simulink model "BLOC_Auxiliary_network_12V"  (R2016a)
settings: Solver=VariableStepAuto  StartTime=0.0  StopTime=10.0  RelTol=1e-3
undefined symbols (not defined in the file): hev_dt, syse_aux_current, syse_aux_voltage, syse_dcdc_efficency, syse_dcdc_in_power
settings Model: Creator=Florent  LastModifiedBy=Florent
settings OptimizationCC: DefaultParameterBehavior=Inlined  OptimizeModelRefInitCode=on  LifeSpan=1
settings RTWCC: SystemTargetFile=ert.tlc  TemplateMakefile=ert_default_tmf  GenerateReport=on  IncludeHyperlinkInReport=on  LaunchReport=on  TargetLang=C++  GenerateTraceInfo=on  GenerateTraceReport=on  GenerateTraceReportSl=on  GenerateTraceReportSf=on  GenerateTraceReportEml=on
settings CodeAppCC: ForceParamTrailComments=on  OperatorAnnotations=on  SimulinkDataObjDesc=on  SFDataObjDesc=on  MATLABFcnDesc=on  InsertBlockDesc=on  MATLABSourceComments=on
settings ERTTargetCC: GenerateSampleERTMain=on  MultiInstanceERTCode=on  CodeInterfacePackaging=C++ class  InlinedParameterPlacement=NonHierarchical  RootIOFormat=Structure reference  ERTCustomFileTemplate=example_file_process.tlc

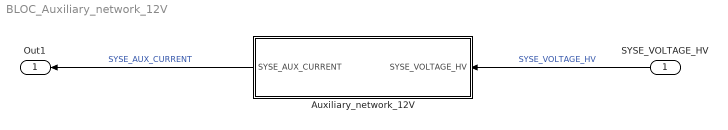
== system BLOC_Auxiliary_network_12V ==
  SYSE_VOLTAGE_HV : Inport
  Auxiliary_network_12V : Subsystem  TreatAsAtomicUnit=on  SystemSampleTime=hev_dt
  Out1 : Outport
  wires:
  Auxiliary_network_12V/1(SYSE_AUX_CURRENT) -> Out1/1  "SYSE_AUX_CURRENT"
  SYSE_VOLTAGE_HV/1 -> Auxiliary_network_12V/1(SYSE_VOLTAGE_HV)  "SYSE_VOLTAGE_HV"

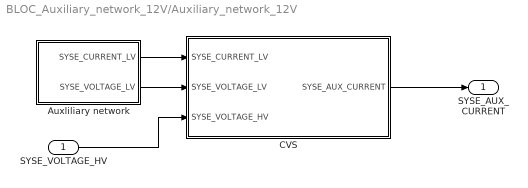
== system BLOC_Auxiliary_network_12V/Auxiliary_network_12V ==
  SYSE_VOLTAGE_HV : Inport
  Auxliliary network : Subsystem
  CVS : Subsystem
  SYSE_AUX_CURRENT : Outport
  wires:
  Auxliliary network/1(SYSE_CURRENT_LV) -> CVS/1(SYSE_CURRENT_LV)
  Auxliliary network/2(SYSE_VOLTAGE_LV) -> CVS/2(SYSE_VOLTAGE_LV)
  CVS/1(SYSE_AUX_CURRENT) -> SYSE_AUX_CURRENT/1
  SYSE_VOLTAGE_HV/1 -> CVS/3(SYSE_VOLTAGE_HV)

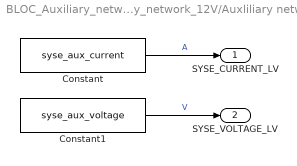
== system BLOC_Auxiliary_network_12V/Auxiliary_network_12V/Auxliliary network ==
  Constant : Constant  Value=syse_aux_current
  Constant1 : Constant  Value=syse_aux_voltage
  SYSE_CURRENT_LV : Outport
  SYSE_VOLTAGE_LV : Outport  Port=2
  wires:
  Constant/1 -> SYSE_CURRENT_LV/1  "A"
  Constant1/1 -> SYSE_VOLTAGE_LV/1  "V"

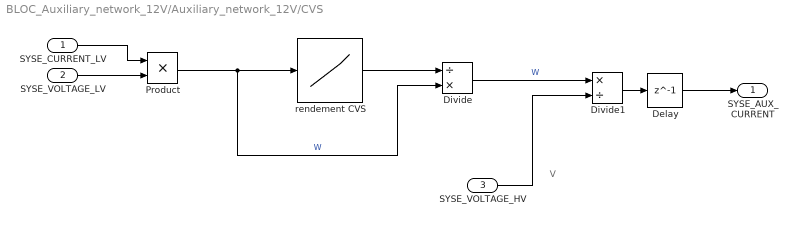
== system BLOC_Auxiliary_network_12V/Auxiliary_network_12V/CVS ==
  note: V
  SYSE_CURRENT_LV : Inport
  SYSE_VOLTAGE_LV : Inport  Port=2
  SYSE_VOLTAGE_HV : Inport  Port=3
  Delay : Delay  DelayLength=1  SampleTime=hev_dt
  Divide : Product  Inputs=/*  SampleTime=hev_dt
  Divide1 : Product  Inputs=*/  SampleTime=hev_dt
  Product : Product  SampleTime=hev_dt  RndMeth=Zero
  rendement CVS : Lookup_n-D  NumberOfTableDimensions=1  BreakpointsForDimension1=syse_dcdc_in_power.*(syse_dcdc_efficency/100)  Table=syse_dcdc_efficency/100  SampleTime=hev_dt  RndMeth=Simplest  InputSameDT=on
  SYSE_AUX_CURRENT : Outport
  wires:
  rendement CVS/1 -> Divide/1
  Divide/1 -> Divide1/1  "W"
  Product/1 -> Divide/2, rendement CVS/1  "W"
  SYSE_VOLTAGE_HV/1 -> Divide1/2
  SYSE_CURRENT_LV/1 -> Product/1
  SYSE_VOLTAGE_LV/1 -> Product/2
  Divide1/1 -> Delay/1
  Delay/1 -> SYSE_AUX_CURRENT/1
